simulink model "AND"  (R2021a)
settings: Solver=FixedStepDiscrete  StartTime=0.0  StopTime=1  FixedStep=1  RelTol=1e-3
settings Model: Creator=KAVITA KUMARI  LastModifiedBy=KAVITA KUMARI
settings OptimizationCC: DefaultParameterBehavior=Inlined  EnhancedBackFolding=on  PassReuseOutputArgsAs=Individual arguments  ZeroExternalMemoryAtStartup=off  ZeroInternalMemoryAtStartup=off  OptimizeBlockOrder=speed  DifferentSizesBufferReuse=on  OptimizationCustomize=off  EfficientTunableParamExpr=on
settings DebuggingCC: ParameterTunabilityLossMsg=error
settings SFSimCC: MATLABDynamicMemAlloc=off
settings RTWCC: SystemTargetFile=ert.tlc  TemplateMakefile=ert_default_tmf
settings CodeAppCC: ForceParamTrailComments=on  IgnoreCustomStorageClasses=off  OperatorAnnotations=on  SimulinkDataObjDesc=on  SFDataObjDesc=on  InsertBlockDesc=on
settings ERTTargetCC: TargetLangStandard=C99 (ISO)  GenerateSampleERTMain=on  InlinedParameterPlacement=NonHierarchical  ERTCustomFileTemplate=example_file_process.tlc

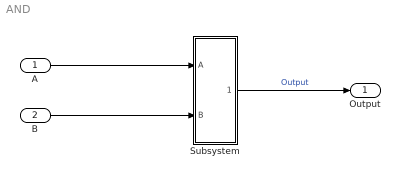
== system AND ==
  A : Inport
  B : Inport  Port=2
  Subsystem : Subsystem  TreatAsAtomicUnit=on
  Output : Outport
  wires:
  A/1 -> Subsystem/1(A)
  B/1 -> Subsystem/2(B)
  Subsystem/1(Output) -> Output/1  "Output"

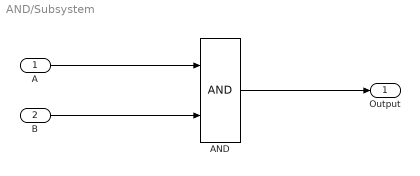
== system AND/Subsystem ==
  A : Inport
  B : Inport  Port=2
  AND : Logic  AllPortsSameDT=off  OutDataTypeStr=boolean
  Output : Outport
  wires:
  A/1 -> AND/1
  B/1 -> AND/2
  AND/1 -> Output/1
